simulink model "DC_Motor_basic_components"  (R2024a)
settings: Solver=FixedStepAuto  StartTime=0.0  StopTime=10.0  FixedStep=25e-6  RelTol=1e-3
model workspace (MAT data in the model file):
  J = 5
  Ke = 1.6
  Kt = 1.3
  L = 0.1
  R = 0.5
  b = 0.01

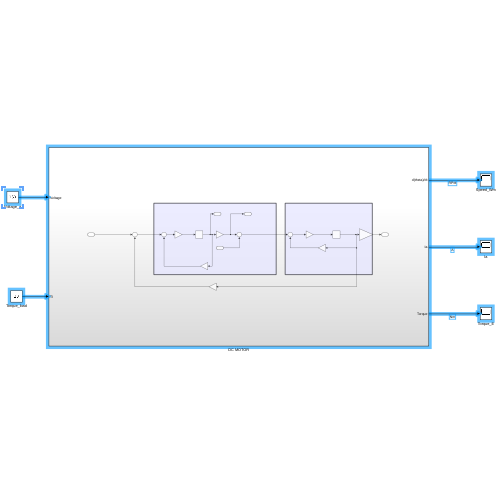
[thumbnail: Simulink's stored preview of the top-level diagram]
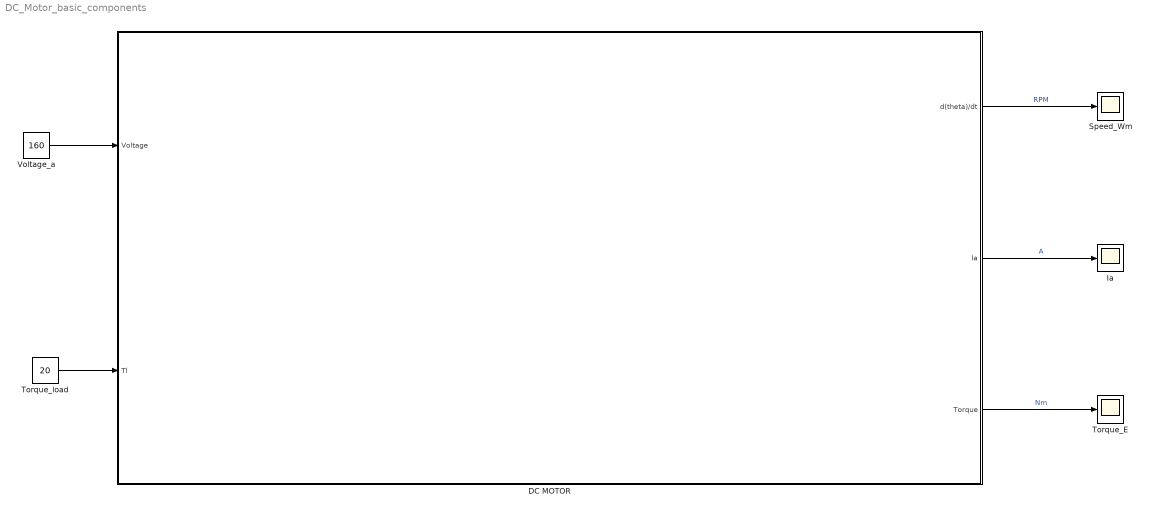
== system DC_Motor_basic_components ==
  DC MOTOR : Subsystem
  Ia : Scope
  Speed_Wm : Scope
  Torque_E : Scope
  Torque_load : Constant  Value=20
  Voltage_a : Constant  Value=160
  wires:
  Voltage_a/1 -> DC MOTOR/1(Voltage)
  DC MOTOR/1(d(theta)/dt) -> Speed_Wm/1  "RPM"
  DC MOTOR/2(Ia) -> Ia/1  "A"
  DC MOTOR/3(Torque) -> Torque_E/1  "Nm"
  Torque_load/1 -> DC MOTOR/2(Tl)

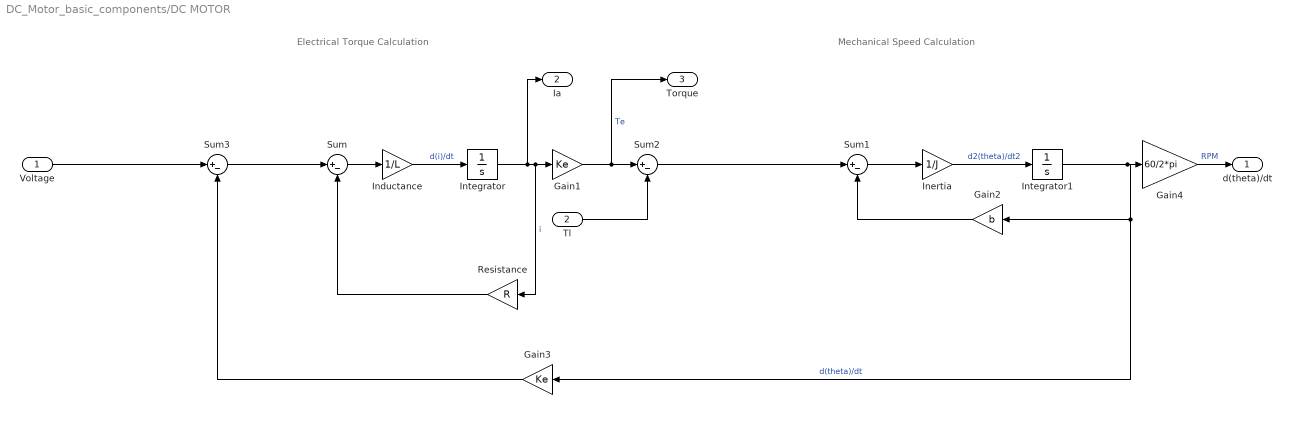
== system DC_Motor_basic_components/DC MOTOR ==
  note: Mechanical Speed Calculation
  note: Electrical Torque Calculation
  Voltage : Inport
  Tl : Inport  Port=2
  Gain1 : Gain  Gain=Ke
  Gain2 : Gain  Gain=b
  Gain3 : Gain  Gain=Ke
  Gain4 : Gain  Gain=60/2*pi
  Inductance : Gain  Gain=1/L
  Inertia : Gain  Gain=1/J
  Integrator : Integrator
  Integrator1 : Integrator
  Resistance : Gain  Gain=R
  Sum{,1..3} (4 alike) : Sum  Inputs=|+-
  d(theta)/dt : Outport
  Ia : Outport  Port=2
  Torque : Outport  Port=3
  wires:
  Inductance/1 -> Integrator/1  "d(i)/dt"
  Sum/1 -> Inductance/1
  Resistance/1 -> Sum/2
  Integrator/1 -> Ia/1, Resistance/1, Gain1/1  "i"
  Gain1/1 -> Sum2/1, Torque/1  "Te"
  Inertia/1 -> Integrator1/1  "d2(theta)/dt2"
  Integrator1/1 -> Gain2/1, Gain3/1, Gain4/1  "d(theta)/dt"
  Sum1/1 -> Inertia/1
  Gain2/1 -> Sum1/2
  Tl/1 -> Sum2/2
  Sum2/1 -> Sum1/1
  Voltage/1 -> Sum3/1
  Sum3/1 -> Sum/1
  Gain3/1 -> Sum3/2
  Gain4/1 -> d(theta)/dt/1  "RPM"
